simulink model "auto_vzmac_core"  (Simulink 7.9)
settings: Solver=ode45  StartTime=0.0  StopTime=2048*16+100  RelTol=1e-3
PreLoadFcn:
  | if ~exist('sync')
  |   sync=[1];
  | end
  | if ~exist('zin0')
  |   zin0=complex( ...
  |     floor(256*rand(1,15*2048+1))/128-1, ...
  |     floor(256*rand(1,15*2048+1))/128-1  ...
  |   );
  | end
undefined symbols (not defined in the file or in its folder): A, B, PCIN, xlipgetpartsetting
libraries: xbsIndex_r4 x23
(part 1 of 4)
settings Model: Creator=mdexter  LastModifiedBy=mdexter

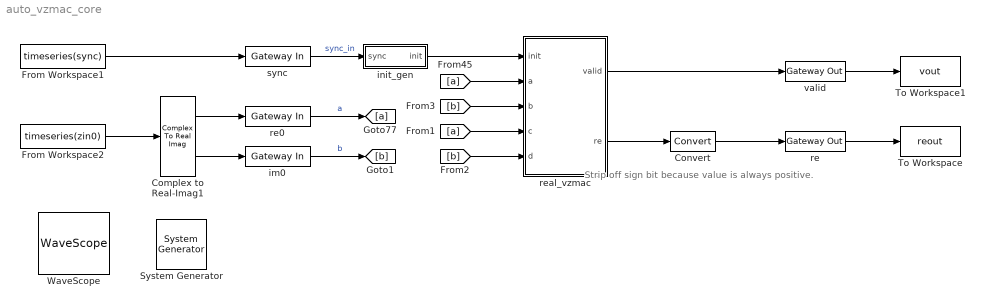
== system auto_vzmac_core ==
  note: Strip off sign bit because
      | value is always positive.
  " System Generator" : xbsIndex_r4/ System Generator  Tag=genX  xilinxfamily=virtex6  part=xc6vsx475t  speed=-1  package=ff1759  synthesis_tool=XST  clock_wrapper=Clock Enables  directory=./auto_vzmac_core  proj_type=Project Navigator  Synth_file=XST Defaults  Impl_file=ISE Defaults  testbench=off  simulink_period=1  sysclk_period=10  dcm_input_clock_period=10  incr_netlist=off  trim_vbits=Everywhere in SubSystem  dbl_ovrd=According to Block Masks  core_generation=According to Block Masks  run_coregen=off  deprecated_control=off  eval_field=0  block_type=sysgen
  Complex to Real-Imag1 : ComplexToRealImag
  Convert : xbsIndex_r4/Convert  gui_display_data_type=Fixed-point  arith_type=Unsigned  n_bits=20  bin_pt=14  float_type=Single  exp_bits=8  fraction_bits=24  quantization=Truncate  overflow=Wrap  en=off  latency=0  dbl_ovrd=off  pipeline=off  block_type=convert
  From Workspace1 : FromWorkspace  VariableName=timeseries(sync)  SampleTime=1  Interpolate=off  OutputAfterFinalValue=Setting to zero
  From Workspace2 : FromWorkspace  VariableName=timeseries(zin0)  SampleTime=1  Interpolate=off  OutputAfterFinalValue=Setting to zero
  To Workspace : ToWorkspace  VariableName=reout  SampleTime=-1
  To Workspace1 : ToWorkspace  VariableName=vout  SampleTime=-1
  WaveScope : xbsIndex_r4/WaveScope  block_type=wavescope
  im0 : xbsIndex_r4/Gateway In  gui_display_data_type=Fixed-point  arith_type="Signed  (2's comp)"  n_bits=8  bin_pt=7  preci_type=Single  exp_width=8  frac_width=24  quantization="Round  (unbiased: +/- Inf)"  overflow=Saturate  period=1  dbl_ovrd=off  timing_constraint=None  locs_specified=off  LOCs={}  UseAsADC=off  ADCChannel='1'  inherit_from_input=off  hdl_port=on  block_type=gatewayin
  init_gen : Subsystem
  re : xbsIndex_r4/Gateway Out  inherit_from_input=off  hdl_port=on  timing_constraint=None  locs_specified=off  LOCs={}  UseAsDAC=off  DACChannel='1'  block_type=gatewayout
      settings: xl_area=[0 0 0 0 21 0 0]
  re0 : xbsIndex_r4/Gateway In  gui_display_data_type=Fixed-point  arith_type="Signed  (2's comp)"  n_bits=8  bin_pt=7  preci_type=Single  exp_width=8  frac_width=24  quantization="Round  (unbiased: +/- Inf)"  overflow=Saturate  period=1  dbl_ovrd=off  timing_constraint=None  locs_specified=off  LOCs={}  UseAsADC=off  ADCChannel='1'  inherit_from_input=off  hdl_port=on  block_type=gatewayin
  real_vzmac : Subsystem
  sync : xbsIndex_r4/Gateway In  gui_display_data_type=Boolean  arith_type=Boolean  n_bits=8  bin_pt=7  preci_type=Single  exp_width=8  frac_width=24  quantization="Round  (unbiased: +/- Inf)"  overflow=Saturate  period=1  dbl_ovrd=off  timing_constraint=None  locs_specified=off  LOCs={}  UseAsADC=off  ADCChannel='1'  inherit_from_input=off  hdl_port=on  block_type=gatewayin
  valid : xbsIndex_r4/Gateway Out  inherit_from_input=off  hdl_port=on  timing_constraint=None  locs_specified=off  LOCs={}  UseAsDAC=off  DACChannel='1'  block_type=gatewayout
      settings: xl_area=[0 0 0 0 21 0 0]
  wires:
  re/1 -> To Workspace/1
  re0/1 -> [a]  "a"
  real_vzmac/1(valid) -> valid/1
  valid/1 -> To Workspace1/1
  real_vzmac/2(re) -> Convert/1
  im0/1 -> [b]  "b"
  [a] -> real_vzmac/2(a)
  [a] -> real_vzmac/4(c)
  [b] -> real_vzmac/3(b)
  [b] -> real_vzmac/5(d)
  From Workspace1/1 -> sync/1
  sync/1 -> init_gen/1(sync)  "sync_in"
  init_gen/1(init) -> real_vzmac/1(init)
  From Workspace2/1 -> Complex to Real-Imag1/1
  Complex to Real-Imag1/1 -> re0/1
  Complex to Real-Imag1/2 -> im0/1
  Convert/1 -> re/1

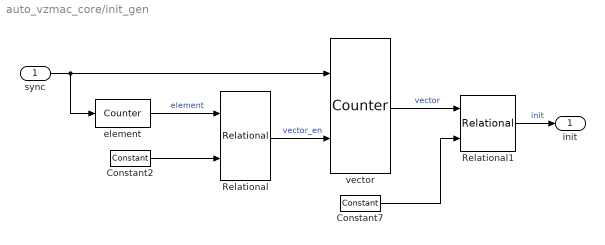
== system auto_vzmac_core/init_gen ==
  sync : Inport
  Constant2 : xbsIndex_r4/Constant  const=2048-2  gui_display_data_type=Fixed-point  arith_type=Unsigned  n_bits=11  bin_pt=0  preci_type=Single  exp_width=8  frac_width=24  explicit_period=on  period=1  equ=P=C  opselect=C  inp2=PCIN>>17  opr=+  inp1=P  carry=CIN  dbl_ovrd=off  block_type=constant
  Constant7 : xbsIndex_r4/Constant  const=0  gui_display_data_type=Fixed-point  arith_type=Unsigned  n_bits=4  bin_pt=0  preci_type=Single  exp_width=8  frac_width=24  explicit_period=on  period=1  equ=P=C  opselect=C  inp2=PCIN>>17  opr=+  inp1=P  carry=CIN  dbl_ovrd=off  block_type=constant
  Relational : xbsIndex_r4/Relational  mode=a=b  en=off  latency=1  dbl_ovrd=off  block_type=relational
  Relational1 : xbsIndex_r4/Relational  mode=a=b  en=off  latency=0  dbl_ovrd=off  block_type=relational
  element : xbsIndex_r4/Counter  cnt_type=Free Running  cnt_to=Inf  operation=Up  start_count=0  cnt_by_val=1  arith_type=Unsigned  n_bits=11  bin_pt=0  load_pin=off  rst=on  en=off  explicit_period=on  period=1  dbl_ovrd=off  use_behavioral_HDL=on  implementation=Fabric  block_type=counter
  vector : xbsIndex_r4/Counter  cnt_type=Count Limited  cnt_to=13  operation=Up  start_count=0  cnt_by_val=1  arith_type=Unsigned  n_bits=4  bin_pt=0  load_pin=off  rst=on  en=on  explicit_period=on  period=1  dbl_ovrd=off  use_behavioral_HDL=on  implementation=Fabric  block_type=counter
  init : Outport
  wires:
  vector/1 -> Relational1/1  "vector"
  Constant7/1 -> Relational1/2
  Constant2/1 -> Relational/2
  Relational/1 -> vector/2  "vector_en"
  element/1 -> Relational/1  "element"
  sync/1 -> vector/1, element/1
  Relational1/1 -> init/1  "init"
